simulink model "pocketcorr2"  (Simulink 6.2)
settings: Solver=ode45  StartTime=0.0  StopTime=1000  RelTol=1e-3
libraries: xbsIndex_r3 x143, xps_library x15, ddc_library x9, cic_library x4, fft_library x3, correlator_library x3, pfb_library x2, delay_lib x1
(part 1 of 2)
settings Model: LastModifiedBy=dejesusc
settings DebuggingCC: SolverPrmCheckMsg=warning

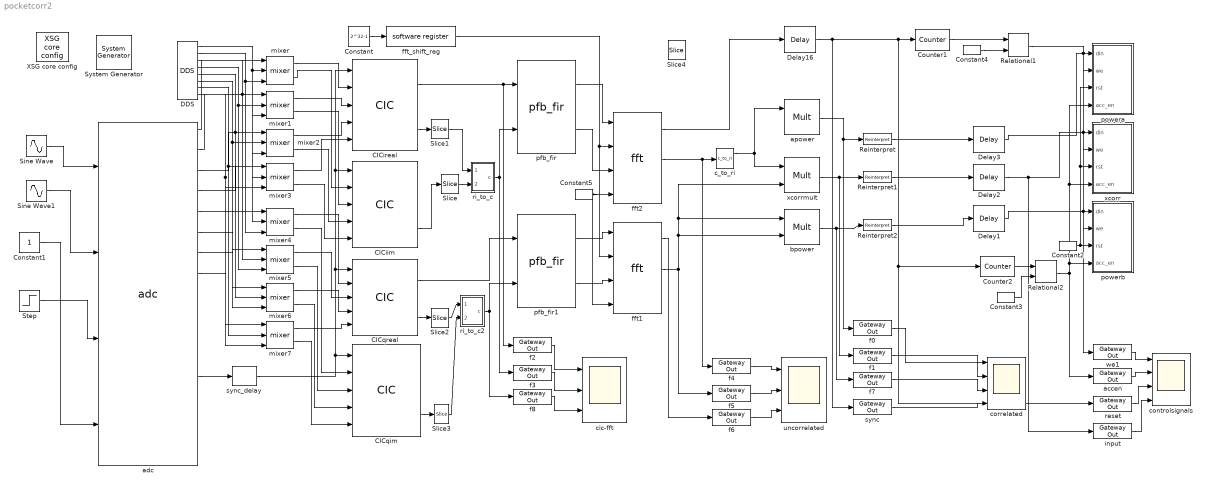
== system pocketcorr2 ==
  " System Generator" : xbsIndex_r3/ System Generator  Tag=genX  xilinxfamily=Virtex2P  part=xc2vp50  speed=-7  package=ff1152  synthesis_tool=XST  directory=./pocketcorr2/sysgen  testbench=off  simulink_period=1  sysclk_period=6.6667  incr_netlist=off  trim_vbits=Everywhere in SubSystem  dbl_ovrd=According to Block Masks  core_generation=According to Block Masks  run_coregen=off  deprecated_control=off  eval_field=0
      settings: AttributesFormatString=System\nGenerator
  CICiim : cic_library/CIC  Description="Cascaded integrator-comb filter.  Linear phase response."  inputs=4  input_bitwidth=16  input_binary_pt=14  D=1  R=1  stages=1  pipeline=off  add_latency=2  int_latency=1  comb_latency=1
  CICireal : cic_library/CIC  Description="Cascaded integrator-comb filter.  Linear phase response."  inputs=4  input_bitwidth=16  input_binary_pt=14  D=1  R=1  stages=1  pipeline=off  add_latency=2  int_latency=1  comb_latency=1
  CICqim : cic_library/CIC  Description="Cascaded integrator-comb filter.  Linear phase response."  inputs=4  input_bitwidth=16  input_binary_pt=14  D=1  R=1  stages=1  pipeline=off  add_latency=2  int_latency=1  comb_latency=1
  CICqreal : cic_library/CIC  Description="Cascaded integrator-comb filter.  Linear phase response."  inputs=4  input_bitwidth=16  input_binary_pt=14  D=1  R=1  stages=1  pipeline=off  add_latency=2  int_latency=1  comb_latency=1
  Constant : Constant  Value=2^32-1
  Constant1 : Constant
  Constant2 : xbsIndex_r3/Constant  const=0  equ=P=C  arith_type=Boolean  n_bits=1  bin_pt=0  opselect=C  inp2=PCIN>>17  opr=+  inp1=P  carry=CIN  iostate=0  explicit_period=on  period=1  dbl_ovrd=off
  Constant3 : xbsIndex_r3/Constant  const=64  equ=P=C  arith_type=Unsigned  n_bits=7  bin_pt=0  opselect=C  inp2=PCIN>>17  opr=+  inp1=P  carry=CIN  iostate=0  explicit_period=on  period=1  dbl_ovrd=off
  Constant4 : xbsIndex_r3/Constant  const=2^4  equ=P=C  arith_type=Unsigned  n_bits=6  bin_pt=0  opselect=C  inp2=PCIN>>17  opr=+  inp1=P  carry=CIN  iostate=0  explicit_period=on  period=1  dbl_ovrd=off
  Constant5 : xbsIndex_r3/Constant  const=0  equ=P=C  arith_type=Unsigned  n_bits=1  bin_pt=0  opselect=C  inp2=PCIN>>17  opr=+  inp1=P  carry=CIN  iostate=0  explicit_period=on  period=1  dbl_ovrd=off
  Counter1 : xbsIndex_r3/Counter  cnt_type=Free Running  n_bits=5  bin_pt=0  arith_type=Unsigned  start_count=0  cnt_to=Inf  cnt_by_val=1  operation=Up  explicit_period=off  period=1  load_pin=off  rst=on  en=off  dbl_ovrd=off  show_param=off  use_rpm=on  gen_core=off
      settings: xl_area=[0, 0, 0, 0, 0, 0, 0]
  Counter2 : xbsIndex_r3/Counter  cnt_type=Free Running  n_bits=8  bin_pt=0  arith_type=Unsigned  start_count=0  cnt_to=Inf  cnt_by_val=1  operation=Up  explicit_period=off  period=1  load_pin=off  rst=on  en=off  dbl_ovrd=off  show_param=off  use_rpm=on  gen_core=off
      settings: xl_area=[0, 0, 0, 0, 0, 0, 0]
  DDS : ddc_library/DDS  freq_div=8  freq=2  num_lo=4  BitWidth=8  latency=2
      link override ddc_lo0/ddc_lo_const/const: equ=P=C
      link override ddc_lo0/ddc_lo_const/const1: equ=P=C
      link override ddc_lo1/ddc_lo_const/const: equ=P=C
      link override ddc_lo1/ddc_lo_const/const1: equ=P=C
      link override ddc_lo2/ddc_lo_const/const: equ=P=C
      link override ddc_lo2/ddc_lo_const/const1: equ=P=C
      link override ddc_lo3/ddc_lo_const/const: equ=P=C
      link override ddc_lo3/ddc_lo_const/const1: equ=P=C
  Delay1 : xbsIndex_r3/Delay  latency=1  reg_retiming=off  explicit_period=on  period=1  en=off  accept_only_valid=off  init_zero=on  dbl_ovrd=off  show_param=off
      settings: xl_area=[0, 0, 0, 0, 0, 0, 0]
  Delay16 : xbsIndex_r3/Delay  latency=5  reg_retiming=off  explicit_period=on  period=1  en=off  accept_only_valid=off  init_zero=on  dbl_ovrd=off  show_param=off
      settings: xl_area=[0, 0, 0, 0, 0, 0, 0]
  Delay2 : xbsIndex_r3/Delay  latency=1  reg_retiming=off  explicit_period=on  period=1  en=off  accept_only_valid=off  init_zero=on  dbl_ovrd=off  show_param=off
      settings: xl_area=[0, 0, 0, 0, 0, 0, 0]
  Delay3 : xbsIndex_r3/Delay  latency=1  reg_retiming=off  explicit_period=on  period=1  en=off  accept_only_valid=off  init_zero=on  dbl_ovrd=off  show_param=off
      settings: xl_area=[0, 0, 0, 0, 0, 0, 0]
  Reinterpret : xbsIndex_r3/Reinterpret  force_arith_type=on  arith_type=Unsigned  force_bin_pt=on  bin_pt=20  force_valid=on
  Reinterpret1 : xbsIndex_r3/Reinterpret  force_arith_type=on  arith_type=Unsigned  force_bin_pt=on  bin_pt=20  force_valid=on
  Reinterpret2 : xbsIndex_r3/Reinterpret  force_arith_type=on  arith_type=Unsigned  force_bin_pt=on  bin_pt=20  force_valid=on
  Relational1 : xbsIndex_r3/Relational  mode=a<b  latency=1  explicit_period=on  period=1  en=off  dbl_ovrd=off  show_param=off
      settings: xl_area=[0, 0, 0, 0, 0, 0, 0]
  Relational2 : xbsIndex_r3/Relational  mode=a<b  latency=1  explicit_period=on  period=1  en=off  dbl_ovrd=off  show_param=off
      settings: xl_area=[0, 0, 0, 0, 0, 0, 0]
  Sine Wave : Sin  SampleTime=0
  Sine Wave1 : Sin  Frequency=2  SampleTime=0
  Slice{,1..4} (5 alike) : xbsIndex_r3/Slice  mode=Upper Bit Location + Width  nbits=9  bit1=0  base1=MSB of Input  bit0=0  base0=LSB of Input  boolean_output=off  explicit_period=off  period=1  dbl_ovrd=off
  Step : Step  Time=10  Before=1  After=0  SampleTime=0
  XSG core config : xps_library/XSG core config  Tag=xps:xsg  hw_sys=iBOB  clk_src=adc0_clk  clk_rate=150  sample_period=1  synthesis_tool=XST  mpc_type=powerpc405
  accen : xbsIndex_r3/Gateway Out  output_type=Double  nbits=8  bin_pt=6  arith_type=Boolean  quantization=Truncate  overflow=Wrap  hdl_port=on  timing_constraint=None  locs_specified=off  LOCs={}  needs_fixed_name=off  show_param=off
      settings: xl_area=[0, 0, 0, 0, 0, 0, 0]
  adc : xps_library/adc  Tag=xps:adc  adc_brd=iBOB:adc0  adc_clk_rate=600  adc_interleave=off  sample_period=1
  apower : xbsIndex_r3/Mult  precision=Full  arith_type="Signed  (2's comp)"  n_bits=8  bin_pt=2  quantization=Truncate  overflow=Wrap  latency=5  explicit_period=on  period=1  en=off  dbl_ovrd=off  show_param=off  mult_type=Parallel  oversample=2  use_embedded=off  pipeline=on  use_rpm=on  placement_style=Rectangular Shape  gen_core=off
      settings: xl_area=[0, 0, 0, 0, 0, 0, 0]
  bpower : xbsIndex_r3/Mult  precision=Full  arith_type="Signed  (2's comp)"  n_bits=8  bin_pt=2  quantization=Truncate  overflow=Wrap  latency=5  explicit_period=on  period=1  en=off  dbl_ovrd=off  show_param=off  mult_type=Parallel  oversample=2  use_embedded=off  pipeline=on  use_rpm=on  placement_style=Rectangular Shape  gen_core=off
      settings: xl_area=[0, 0, 0, 0, 0, 0, 0]
  c_to_ri : fft_library/c_to_ri  BitWidth=18
  cic-fft : Scope  NumInputPorts=3
      settings: YMin=-5~-5~-5  YMax=5~5~5  SaveName=ScopeData3
  controlsignals : Scope  NumInputPorts=4
      settings: YMin=-5~-5~-5~-5  YMax=5~5~5~5  SaveName=ScopeData4
  correlated : Scope  NumInputPorts=4
      settings: YMin=-5~-5~-5~-5  YMax=5~5~5~5
  f{0..1,3..8} (8 alike) : xbsIndex_r3/Gateway Out  output_type=Double  nbits=8  bin_pt=6  arith_type=Boolean  quantization=Truncate  overflow=Wrap  hdl_port=on  timing_constraint=None  locs_specified=off  LOCs={}  needs_fixed_name=off  show_param=off
      settings: xl_area=[0, 0, 0, 0, 0, 0, 0]
  f2 : xbsIndex_r3/Gateway Out  output_type=Automatic  nbits=8  bin_pt=6  arith_type=Boolean  quantization=Truncate  overflow=Wrap  hdl_port=on  timing_constraint=None  locs_specified=off  LOCs={}  needs_fixed_name=off  show_param=off
      settings: xl_area=[0, 0, 0, 0, 0, 0, 0]
  fft1 : fft_library/fft  FFTSize=5  BitWidth=72  n_inputs=0  quantization=Truncate  overflow=Wrap  add_latency=2  mult_latency=3  bram_latency=2
  fft2 : fft_library/fft  FFTSize=5  BitWidth=72  n_inputs=0  quantization=Truncate  overflow=Wrap  add_latency=2  mult_latency=3  bram_latency=2
  fft_shift_reg : xps_library/software register  Tag=xps:sw_reg  io_dir=From Processor  arith_type=Unsigned  bitwidth=32  bin_pt=0  sample_period=1  gw_name=pocketcorr2_fft_shift_reg_user_data_out
  input : xbsIndex_r3/Gateway Out  output_type=Double  nbits=8  bin_pt=6  arith_type=Boolean  quantization=Truncate  overflow=Wrap  hdl_port=on  timing_constraint=None  locs_specified=off  LOCs={}  needs_fixed_name=off  show_param=off
      settings: xl_area=[0, 0, 0, 0, 0, 0, 0]
  mixer{,1..7} (8 alike) : ddc_library/mixer  BitWidth=18  latency=2
  pfb_fir : pfb_library/pfb_fir  PFBSize=5  TotalTaps=2  WindowType=hamming  n_inputs=0  MakeBiplex=off  BitWidthIn=18  BitWidthOut=36  CoeffBitWidth=8  CoeffDistMem=off  add_latency=2  mult_latency=3  bram_latency=2  quantization="Round  (unbiased: +/- Inf)"  fwidth=1
      link override pol1_in1_first_tap/sync_delay/Constant: equ=P=C
      link override pol1_in1_first_tap/sync_delay/Constant1: equ=P=C
      link override pol1_in1_first_tap/sync_delay/Constant2: equ=P=C
      link override pol1_in1_first_tap/sync_delay/Constant3: equ=P=C
  pfb_fir1 : pfb_library/pfb_fir  PFBSize=5  TotalTaps=2  WindowType=hamming  n_inputs=0  MakeBiplex=off  BitWidthIn=18  BitWidthOut=36  CoeffBitWidth=8  CoeffDistMem=off  add_latency=2  mult_latency=3  bram_latency=2  quantization="Round  (unbiased: +/- Inf)"  fwidth=1
      link override pol1_in1_first_tap/sync_delay/Constant: equ=P=C
      link override pol1_in1_first_tap/sync_delay/Constant1: equ=P=C
      link override pol1_in1_first_tap/sync_delay/Constant2: equ=P=C
      link override pol1_in1_first_tap/sync_delay/Constant3: equ=P=C
  powera : Subsystem  AncestorBlock=correlator_library/vacc  mask{vlen=32/2-1, n_bits=32, bin_pt=0, add_latency=2, arith_type=Unsigned, BitWidthIn=72, BinPtIn=20, streams=1}
      mask prompts: vlen "Vector Length"; n_bits "Output Sample Bit Width"; bin_pt "Output Binary Point"; add_latency "Add Latency"; arith_type "Arithmetic Type"; BitWidthIn "Input Bit Width"; BinPtIn "Input Binary Point"; streams "Number of Parallel Streams"
      mask init:
      | cursys = gcb;
      | disp(cursys);
      | 
      | core = [cursys,'/acc_core'];
      | if ~strcmp(get_param(core, 'arith_type'), arith_type),
      |     set_param(core, 'arith_type', arith_type);
      | end
      mask StyleString: edit,edit,edit,edit,popup(Unsigned|Signed  (2's comp)),edit,edit,edit
  powerb : Subsystem  AncestorBlock=correlator_library/vacc  mask{vlen=32/2-1, n_bits=32, bin_pt=0, add_latency=2, arith_type=Unsigned, BitWidthIn=72, BinPtIn=20, streams=1}
      mask prompts: vlen "Vector Length"; n_bits "Output Sample Bit Width"; bin_pt "Output Binary Point"; add_latency "Add Latency"; arith_type "Arithmetic Type"; BitWidthIn "Input Bit Width"; BinPtIn "Input Binary Point"; streams "Number of Parallel Streams"
      mask init:
      | cursys = gcb;
      | disp(cursys);
      | 
      | core = [cursys,'/acc_core'];
      | if ~strcmp(get_param(core, 'arith_type'), arith_type),
      |     set_param(core, 'arith_type', arith_type);
      | end
      mask StyleString: edit,edit,edit,edit,popup(Unsigned|Signed  (2's comp)),edit,edit,edit
  reset : xbsIndex_r3/Gateway Out  output_type=Double  nbits=8  bin_pt=6  arith_type=Boolean  quantization=Truncate  overflow=Wrap  hdl_port=on  timing_constraint=None  locs_specified=off  LOCs={}  needs_fixed_name=off  show_param=off
      settings: xl_area=[0, 0, 0, 0, 0, 0, 0]
  ri_to_c : Subsystem  AncestorBlock=fft_library/ri_to_c  mask{likes_cookies=on}
      mask prompts: likes_cookies "I think cookies are delicious"
  ri_to_c2 : Subsystem  AncestorBlock=fft_library/ri_to_c  mask{likes_cookies=on}
      mask prompts: likes_cookies "I think cookies are delicious"
  sync : xbsIndex_r3/Gateway Out  output_type=Double  nbits=8  bin_pt=6  arith_type=Boolean  quantization=Truncate  overflow=Wrap  hdl_port=on  timing_constraint=None  locs_specified=off  LOCs={}  needs_fixed_name=off  show_param=off
      settings: xl_area=[0, 0, 0, 0, 0, 0, 0]
  sync_delay : delay_lib/sync_delay  DelayLen=4
      link override Constant: equ=P=C
      link override Constant1: equ=P=C
      link override Constant2: equ=P=C
      link override Constant3: equ=P=C
  uncorrelated : Scope  NumInputPorts=3
      settings: YMin=-5~-5~-5  YMax=5~5~5  SaveName=ScopeData2
  we1 : xbsIndex_r3/Gateway Out  output_type=Double  nbits=8  bin_pt=6  arith_type=Boolean  quantization=Truncate  overflow=Wrap  hdl_port=on  timing_constraint=None  locs_specified=off  LOCs={}  needs_fixed_name=off  show_param=off
      settings: xl_area=[0, 0, 0, 0, 0, 0, 0]
  xcorr : Subsystem  AncestorBlock=correlator_library/vacc  mask{vlen=32/2-1, n_bits=32, bin_pt=0, add_latency=2, arith_type=Unsigned, BitWidthIn=72, BinPtIn=20, streams=1}
      mask prompts: vlen "Vector Length"; n_bits "Output Sample Bit Width"; bin_pt "Output Binary Point"; add_latency "Add Latency"; arith_type "Arithmetic Type"; BitWidthIn "Input Bit Width"; BinPtIn "Input Binary Point"; streams "Number of Parallel Streams"
      mask init:
      | cursys = gcb;
      | disp(cursys);
      | 
      | core = [cursys,'/acc_core'];
      | if ~strcmp(get_param(core, 'arith_type'), arith_type),
      |     set_param(core, 'arith_type', arith_type);
      | end
      mask StyleString: edit,edit,edit,edit,popup(Unsigned|Signed  (2's comp)),edit,edit,edit
  xcorrmult : xbsIndex_r3/Mult  precision=Full  arith_type="Signed  (2's comp)"  n_bits=8  bin_pt=2  quantization=Truncate  overflow=Wrap  latency=5  explicit_period=on  period=1  en=off  dbl_ovrd=off  show_param=off  mult_type=Parallel  oversample=2  use_embedded=off  pipeline=on  use_rpm=on  placement_style=Rectangular Shape  gen_core=off
      settings: xl_area=[0, 0, 0, 0, 0, 0, 0]
  wires:
  Constant/1 -> fft_shift_reg/1
  Constant1/1 -> adc/4
  apower/1 -> f0/1, Reinterpret/1
  xcorrmult/1 -> f1/1, Reinterpret1/1
  Delay16/1 -> Counter1/1, Counter2/1, reset/1, sync/1
  Step/1 -> adc/3
  Sine Wave/1 -> adc/1
  Counter1/1 -> Relational1/1
  Constant4/1 -> Relational1/2
  Relational1/1 -> powera/2(we), powerb/2(we), we1/1, xcorr/2(we)
  Constant2/1 -> powerb/3(rst), xcorr/3(rst), powera/3(rst)
  Relational2/1 -> accen/1, powerb/4(acc_en), xcorr/4(acc_en), powera/4(acc_en)
  Counter2/1 -> Relational2/1
  Constant3/1 -> Relational2/2
  f0/1 -> correlated/1
  f1/1 -> correlated/2
  f4/1 -> uncorrelated/1
  f5/1 -> uncorrelated/2
  f6/1 -> uncorrelated/3
  DDS/1 -> mixer/2, mixer4/2
  DDS/2 -> mixer/3, mixer4/3
  adc/1 -> mixer/1
  DDS/3 -> mixer1/2, mixer5/2
  DDS/4 -> mixer1/3, mixer5/3
  DDS/5 -> mixer2/2, mixer6/2
  DDS/6 -> mixer2/3, mixer6/3
  adc/2 -> mixer1/1
  adc/3 -> mixer2/1
  adc/4 -> mixer3/1
  adc/5 -> mixer4/1
  adc/6 -> mixer5/1
  adc/7 -> mixer6/1
  adc/8 -> mixer7/1
  DDS/7 -> mixer3/2, mixer7/2
  DDS/8 -> mixer3/3, mixer7/3
  adc/13 -> sync_delay/1
  bpower/1 -> Reinterpret2/1, f7/1
  fft_shift_reg/1 -> fft2/2, fft1/2
  fft2/1 -> Delay16/1
  fft1/2 -> xcorrmult/2, bpower/1, bpower/2, f5/1
  fft2/2 -> f4/1, c_to_ri/1
  fft1/1 -> f6/1
  sync/1 -> correlated/4
  f7/1 -> correlated/3
  CICireal/2 -> Slice1/1
  CICiim/2 -> Slice/1
  CICqreal/2 -> Slice2/1
  CICqim/2 -> Slice3/1
  ri_to_c2/1(c) -> f8/1, pfb_fir1/2
  ri_to_c/1(c) -> f3/1, pfb_fir/2
  CICireal/1 -> f2/1, pfb_fir/1
  f2/1 -> cic-fft/1
  f3/1 -> cic-fft/2
  f8/1 -> cic-fft/3
  Constant5/1 -> fft2/4, fft1/4
  Slice/1 -> ri_to_c/2(im)
  Slice1/1 -> ri_to_c/1(re)
  Slice2/1 -> ri_to_c2/1(re)
  Slice3/1 -> ri_to_c2/2(im)
  we1/1 -> controlsignals/1
  accen/1 -> controlsignals/2
  reset/1 -> controlsignals/3
  input/1 -> controlsignals/4
  Delay1/1 -> powerb/1(din)
  Reinterpret/1 -> Delay3/1
  Reinterpret1/1 -> Delay2/1
  Reinterpret2/1 -> Delay1/1
  Delay2/1 -> xcorr/1(din), input/1
  Delay3/1 -> powera/1(din)
  sync_delay/1 -> CICqim/1, CICqreal/1, CICiim/1, CICireal/1
  mixer/1 -> CICireal/2
  mixer/2 -> CICiim/2
  mixer1/1 -> CICireal/3
  mixer1/2 -> CICiim/3
  mixer2/1 -> CICireal/4
  mixer2/2 -> CICiim/4
  mixer3/1 -> CICireal/5
  mixer3/2 -> CICiim/5
  mixer4/1 -> CICqreal/2
  mixer5/1 -> CICqreal/3
  mixer6/1 -> CICqreal/4
  mixer7/1 -> CICqreal/5
  mixer4/2 -> CICqim/2
  mixer5/2 -> CICqim/3
  mixer6/2 -> CICqim/4
  mixer7/2 -> CICqim/5
  pfb_fir1/2 -> fft1/3
  pfb_fir1/1 -> fft1/1
  CICqreal/1 -> pfb_fir1/1
  pfb_fir/2 -> fft2/3
  pfb_fir/1 -> fft2/1
  Sine Wave1/1 -> adc/2
  c_to_ri/1 -> apower/1, xcorrmult/1

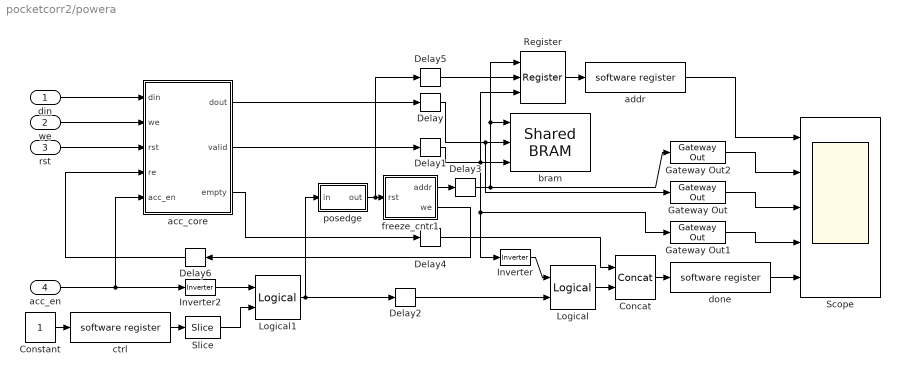
== system pocketcorr2/powera ==
  din : Inport  Port=1  LatchInput=off
  we : Inport  Port=2  LatchInput=off
  rst : Inport  Port=3  LatchInput=off
  acc_en : Inport  Port=4  LatchInput=off
  Concat : xbsIndex_r3/Concat  num_inputs=2  explicit_period=off  period=1  dbl_ovrd=off
  Constant : Constant
  Delay : xbsIndex_r3/Delay  latency=1  reg_retiming=off  explicit_period=off  period=1  en=off  accept_only_valid=off  init_zero=on  dbl_ovrd=off  show_param=off
      settings: xl_area=[0, 0, 0, 0, 0, 0, 0]
  Delay1 : xbsIndex_r3/Delay  latency=1  reg_retiming=off  explicit_period=off  period=1  en=off  accept_only_valid=off  init_zero=on  dbl_ovrd=off  show_param=off
      settings: xl_area=[0, 0, 0, 0, 0, 0, 0]
  Delay2 : xbsIndex_r3/Delay  latency=6  reg_retiming=off  explicit_period=off  period=1  en=off  accept_only_valid=off  init_zero=on  dbl_ovrd=off  show_param=off
      settings: xl_area=[0, 0, 0, 0, 0, 0, 0]
  Delay3 : xbsIndex_r3/Delay  latency=4  reg_retiming=off  explicit_period=off  period=1  en=off  accept_only_valid=off  init_zero=on  dbl_ovrd=off  show_param=off
      settings: xl_area=[0, 0, 0, 0, 0, 0, 0]
  Delay4 : xbsIndex_r3/Delay  latency=2  reg_retiming=off  explicit_period=on  period=1  en=off  accept_only_valid=off  init_zero=on  dbl_ovrd=off  show_param=off
      settings: xl_area=[0, 0, 0, 0, 0, 0, 0]
  Delay5 : xbsIndex_r3/Delay  latency=3  reg_retiming=off  explicit_period=off  period=1  en=off  accept_only_valid=off  init_zero=on  dbl_ovrd=off  show_param=off
      settings: xl_area=[0, 0, 0, 0, 0, 0, 0]
  Delay6 : xbsIndex_r3/Delay  Orientation=left  latency=3  reg_retiming=off  explicit_period=off  period=1  en=off  accept_only_valid=off  init_zero=on  dbl_ovrd=off  show_param=off
      settings: xl_area=[0, 0, 0, 0, 0, 0, 0]
  Gateway Out : xbsIndex_r3/Gateway Out  output_type=Double  nbits=8  bin_pt=6  arith_type=Boolean  quantization=Truncate  overflow=Wrap  hdl_port=off  timing_constraint=None  locs_specified=off  LOCs={}  needs_fixed_name=off  show_param=off
      settings: xl_area=[0, 0, 0, 0, 0, 0, 0]
  Gateway Out1 : xbsIndex_r3/Gateway Out  output_type=Double  nbits=8  bin_pt=6  arith_type=Boolean  quantization=Truncate  overflow=Wrap  hdl_port=off  timing_constraint=None  locs_specified=off  LOCs={}  needs_fixed_name=off  show_param=off
      settings: xl_area=[0, 0, 0, 0, 0, 0, 0]
  Gateway Out2 : xbsIndex_r3/Gateway Out  output_type=Double  nbits=8  bin_pt=6  arith_type=Boolean  quantization=Truncate  overflow=Wrap  hdl_port=off  timing_constraint=None  locs_specified=off  LOCs={}  needs_fixed_name=off  show_param=off
      settings: xl_area=[0, 0, 0, 0, 0, 0, 0]
  Inverter : xbsIndex_r3/Inverter  latency=0  explicit_period=off  period=1  en=off  dbl_ovrd=off  show_param=off
      settings: xl_area=[0, 0, 0, 0, 0, 0, 0]
  Inverter2 : xbsIndex_r3/Inverter  latency=0  explicit_period=off  period=1  en=off  dbl_ovrd=off  show_param=off
      settings: xl_area=[0, 0, 0, 0, 0, 0, 0]
  Logical : xbsIndex_r3/Logical  logical_function=AND  inputs=2  precision=Full  arith_type=Unsigned  n_bits=8  bin_pt=2  align_bp=on  latency=0  explicit_period=off  period=1  en=off  dbl_ovrd=off  show_param=off
      settings: xl_area=[0, 0, 0, 0, 0, 0, 0]
  Logical1 : xbsIndex_r3/Logical  logical_function=AND  inputs=2  precision=Full  arith_type=Unsigned  n_bits=8  bin_pt=2  align_bp=on  latency=1  explicit_period=off  period=1  en=off  dbl_ovrd=off  show_param=off
      settings: xl_area=[0, 0, 0, 0, 0, 0, 0]
  Register : xbsIndex_r3/Register  init=0  reg_only_valid=off  explicit_period=off  period=1  rst=on  en=on  out_en=off  dbl_ovrd=off  show_param=off
      settings: xl_area=[0, 0, 0, 0, 0, 0, 0]
  Scope : Scope  NumInputPorts=5
      settings: YMin=0~0~0~0~0  YMax=50~200~4~1~3
  Slice : xbsIndex_r3/Slice  mode=Lower Bit Location + Width  nbits=1  bit1=0  base1=MSB of Input  bit0=0  base0=LSB of Input  boolean_output=on  explicit_period=off  period=1  dbl_ovrd=off
  acc_core : Subsystem  mask{vlen=vlen, n_bits=n_bits, bin_pt=bin_pt, add_latency=add_latency, arith_type=Unsigned, BitWidthIn=BitWidthIn, BinPtIn=BinPtIn, streams=streams}
      mask prompts: vlen "Vector Length"; n_bits "Output Sample Bit Width"; bin_pt "Output Binary Point"; add_latency "Add Latency"; arith_type "Arithmetic Type"; BitWidthIn "Input Bit Width"; BinPtIn "Input Binary Point"; streams "Number of Parallel Streams"
      mask init:
      | acc_core_mask;
      mask StyleString: edit,edit,edit,edit,popup(Unsigned|Signed  (2's comp)),edit,edit,edit
  addr : xps_library/software register  Tag=xps:sw_reg  io_dir=To Processor  arith_type=Unsigned  bitwidth=32  bin_pt=0  sample_period=1  gw_name=pocketcorr2_powera_addr_user_data_in
  bram : xps_library/Shared BRAM  Tag=xps:bram  arith_type="Signed  (2's comp)"  addr_width=11  data_width=32  data_bin_pt=bin_pt  init_vals=0  sample_rate=1
  ctrl : xps_library/software register  Tag=xps:sw_reg  io_dir=From Processor  arith_type=Unsigned  bitwidth=32  bin_pt=0  sample_period=1  gw_name=pocketcorr2_powera_ctrl_user_data_out
  done : xps_library/software register  Tag=xps:sw_reg  io_dir=To Processor  arith_type=Unsigned  bitwidth=32  bin_pt=0  sample_period=1  gw_name=pocketcorr2_powera_done_user_data_in
  freeze_cntr1 : Subsystem  mask{CounterBits=11}
      mask prompts: CounterBits "Counter Length (2^?)"
  posedge : Subsystem
  wires:
  Delay5/1 -> Register/2
  Delay6/1 -> acc_core/4(re)
  Delay4/1 -> Concat/1
  Concat/1 -> done/1
  Logical/1 -> Concat/2
  acc_core/3(empty) -> Delay4/1
  Register/1 -> addr/1
  Delay3/1 -> Register/1, bram/1, Gateway Out2/1
  Delay2/1 -> Logical/2
  Delay1/1 -> Register/3, bram/3, Inverter/1, Gateway Out1/1
  Constant/1 -> ctrl/1
  Delay/1 -> Gateway Out/1, bram/2
  din/1 -> acc_core/1(din)
  we/1 -> acc_core/2(we)
  rst/1 -> acc_core/3(rst)
  acc_core/2(valid) -> Delay1/1
  freeze_cntr1/1(addr) -> Delay3/1
  freeze_cntr1/2(we) -> Delay6/1
  acc_core/1(dout) -> Delay/1
  Inverter/1 -> Logical/1
  acc_en/1 -> acc_core/5(acc_en), Inverter2/1
  ctrl/1 -> Slice/1
  Slice/1 -> Logical1/2
  Inverter2/1 -> Logical1/1
  Logical1/1 -> Delay2/1, posedge/1(in)
  posedge/1(out) -> Delay5/1, freeze_cntr1/1(rst)
  done/1 -> Scope/5
  Gateway Out1/1 -> Scope/4
  Gateway Out/1 -> Scope/3
  addr/1 -> Scope/1
  Gateway Out2/1 -> Scope/2

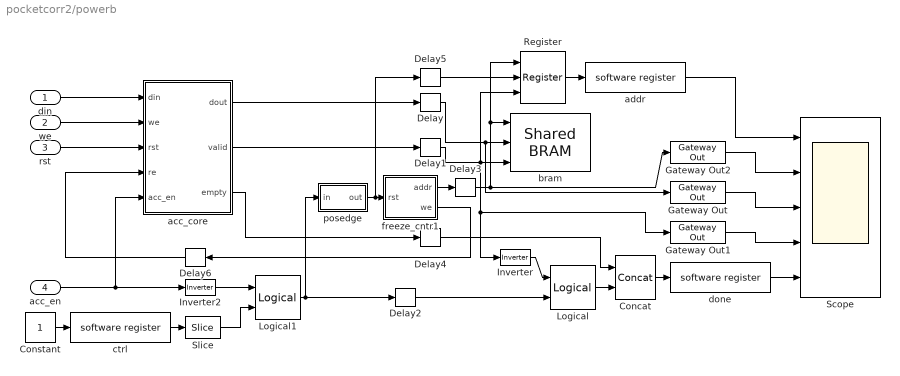
== system pocketcorr2/powerb ==
  din : Inport  Port=1  LatchInput=off
  we : Inport  Port=2  LatchInput=off
  rst : Inport  Port=3  LatchInput=off
  acc_en : Inport  Port=4  LatchInput=off
  Concat : xbsIndex_r3/Concat  num_inputs=2  explicit_period=off  period=1  dbl_ovrd=off
  Constant : Constant
  Delay : xbsIndex_r3/Delay  latency=1  reg_retiming=off  explicit_period=off  period=1  en=off  accept_only_valid=off  init_zero=on  dbl_ovrd=off  show_param=off
      settings: xl_area=[0, 0, 0, 0, 0, 0, 0]
  Delay1 : xbsIndex_r3/Delay  latency=1  reg_retiming=off  explicit_period=off  period=1  en=off  accept_only_valid=off  init_zero=on  dbl_ovrd=off  show_param=off
      settings: xl_area=[0, 0, 0, 0, 0, 0, 0]
  Delay2 : xbsIndex_r3/Delay  latency=6  reg_retiming=off  explicit_period=off  period=1  en=off  accept_only_valid=off  init_zero=on  dbl_ovrd=off  show_param=off
      settings: xl_area=[0, 0, 0, 0, 0, 0, 0]
  Delay3 : xbsIndex_r3/Delay  latency=4  reg_retiming=off  explicit_period=off  period=1  en=off  accept_only_valid=off  init_zero=on  dbl_ovrd=off  show_param=off
      settings: xl_area=[0, 0, 0, 0, 0, 0, 0]
  Delay4 : xbsIndex_r3/Delay  latency=2  reg_retiming=off  explicit_period=on  period=1  en=off  accept_only_valid=off  init_zero=on  dbl_ovrd=off  show_param=off
      settings: xl_area=[0, 0, 0, 0, 0, 0, 0]
  Delay5 : xbsIndex_r3/Delay  latency=3  reg_retiming=off  explicit_period=off  period=1  en=off  accept_only_valid=off  init_zero=on  dbl_ovrd=off  show_param=off
      settings: xl_area=[0, 0, 0, 0, 0, 0, 0]
  Delay6 : xbsIndex_r3/Delay  Orientation=left  latency=3  reg_retiming=off  explicit_period=off  period=1  en=off  accept_only_valid=off  init_zero=on  dbl_ovrd=off  show_param=off
      settings: xl_area=[0, 0, 0, 0, 0, 0, 0]
  Gateway Out : xbsIndex_r3/Gateway Out  output_type=Double  nbits=8  bin_pt=6  arith_type=Boolean  quantization=Truncate  overflow=Wrap  hdl_port=off  timing_constraint=None  locs_specified=off  LOCs={}  needs_fixed_name=off  show_param=off
      settings: xl_area=[0, 0, 0, 0, 0, 0, 0]
  Gateway Out1 : xbsIndex_r3/Gateway Out  output_type=Double  nbits=8  bin_pt=6  arith_type=Boolean  quantization=Truncate  overflow=Wrap  hdl_port=off  timing_constraint=None  locs_specified=off  LOCs={}  needs_fixed_name=off  show_param=off
      settings: xl_area=[0, 0, 0, 0, 0, 0, 0]
  Gateway Out2 : xbsIndex_r3/Gateway Out  output_type=Double  nbits=8  bin_pt=6  arith_type=Boolean  quantization=Truncate  overflow=Wrap  hdl_port=off  timing_constraint=None  locs_specified=off  LOCs={}  needs_fixed_name=off  show_param=off
      settings: xl_area=[0, 0, 0, 0, 0, 0, 0]
  Inverter : xbsIndex_r3/Inverter  latency=0  explicit_period=off  period=1  en=off  dbl_ovrd=off  show_param=off
      settings: xl_area=[0, 0, 0, 0, 0, 0, 0]
  Inverter2 : xbsIndex_r3/Inverter  latency=0  explicit_period=off  period=1  en=off  dbl_ovrd=off  show_param=off
      settings: xl_area=[0, 0, 0, 0, 0, 0, 0]
  Logical : xbsIndex_r3/Logical  logical_function=AND  inputs=2  precision=Full  arith_type=Unsigned  n_bits=8  bin_pt=2  align_bp=on  latency=0  explicit_period=off  period=1  en=off  dbl_ovrd=off  show_param=off
      settings: xl_area=[0, 0, 0, 0, 0, 0, 0]
  Logical1 : xbsIndex_r3/Logical  logical_function=AND  inputs=2  precision=Full  arith_type=Unsigned  n_bits=8  bin_pt=2  align_bp=on  latency=1  explicit_period=off  period=1  en=off  dbl_ovrd=off  show_param=off
      settings: xl_area=[0, 0, 0, 0, 0, 0, 0]
  Register : xbsIndex_r3/Register  init=0  reg_only_valid=off  explicit_period=off  period=1  rst=on  en=on  out_en=off  dbl_ovrd=off  show_param=off
      settings: xl_area=[0, 0, 0, 0, 0, 0, 0]
  Scope : Scope  NumInputPorts=5
      settings: YMin=0~0~0~0~0  YMax=50~200~4~1~3
  Slice : xbsIndex_r3/Slice  mode=Lower Bit Location + Width  nbits=1  bit1=0  base1=MSB of Input  bit0=0  base0=LSB of Input  boolean_output=on  explicit_period=off  period=1  dbl_ovrd=off
  acc_core : Subsystem  mask{vlen=vlen, n_bits=n_bits, bin_pt=bin_pt, add_latency=add_latency, arith_type=Unsigned, BitWidthIn=BitWidthIn, BinPtIn=BinPtIn, streams=streams}
      mask prompts: vlen "Vector Length"; n_bits "Output Sample Bit Width"; bin_pt "Output Binary Point"; add_latency "Add Latency"; arith_type "Arithmetic Type"; BitWidthIn "Input Bit Width"; BinPtIn "Input Binary Point"; streams "Number of Parallel Streams"
      mask init:
      | acc_core_mask;
      mask StyleString: edit,edit,edit,edit,popup(Unsigned|Signed  (2's comp)),edit,edit,edit
  addr : xps_library/software register  Tag=xps:sw_reg  io_dir=To Processor  arith_type=Unsigned  bitwidth=32  bin_pt=0  sample_period=1  gw_name=pocketcorr2_powerb_addr_user_data_in
  bram : xps_library/Shared BRAM  Tag=xps:bram  arith_type="Signed  (2's comp)"  addr_width=11  data_width=32  data_bin_pt=bin_pt  init_vals=0  sample_rate=1
  ctrl : xps_library/software register  Tag=xps:sw_reg  io_dir=From Processor  arith_type=Unsigned  bitwidth=32  bin_pt=0  sample_period=1  gw_name=pocketcorr2_powerb_ctrl_user_data_out
  done : xps_library/software register  Tag=xps:sw_reg  io_dir=To Processor  arith_type=Unsigned  bitwidth=32  bin_pt=0  sample_period=1  gw_name=pocketcorr2_powerb_done_user_data_in
  freeze_cntr1 : Subsystem  mask{CounterBits=11}
      mask prompts: CounterBits "Counter Length (2^?)"
  posedge : Subsystem
  wires:
  Delay5/1 -> Register/2
  Delay6/1 -> acc_core/4(re)
  Delay4/1 -> Concat/1
  Concat/1 -> done/1
  Logical/1 -> Concat/2
  acc_core/3(empty) -> Delay4/1
  Register/1 -> addr/1
  Delay3/1 -> Register/1, bram/1, Gateway Out2/1
  Delay2/1 -> Logical/2
  Delay1/1 -> Register/3, bram/3, Inverter/1, Gateway Out1/1
  Constant/1 -> ctrl/1
  Delay/1 -> Gateway Out/1, bram/2
  din/1 -> acc_core/1(din)
  we/1 -> acc_core/2(we)
  rst/1 -> acc_core/3(rst)
  acc_core/2(valid) -> Delay1/1
  freeze_cntr1/1(addr) -> Delay3/1
  freeze_cntr1/2(we) -> Delay6/1
  acc_core/1(dout) -> Delay/1
  Inverter/1 -> Logical/1
  acc_en/1 -> acc_core/5(acc_en), Inverter2/1
  ctrl/1 -> Slice/1
  Slice/1 -> Logical1/2
  Inverter2/1 -> Logical1/1
  Logical1/1 -> Delay2/1, posedge/1(in)
  posedge/1(out) -> Delay5/1, freeze_cntr1/1(rst)
  done/1 -> Scope/5
  Gateway Out1/1 -> Scope/4
  Gateway Out/1 -> Scope/3
  addr/1 -> Scope/1
  Gateway Out2/1 -> Scope/2

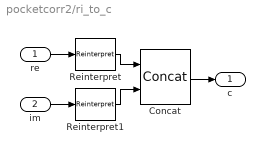
== system pocketcorr2/ri_to_c ==
  re : Inport  Port=1  LatchInput=off
  im : Inport  Port=2  LatchInput=off
  Concat : xbsIndex_r3/Concat  num_inputs=2  explicit_period=on  period=1  dbl_ovrd=off
  Reinterpret : xbsIndex_r3/Reinterpret  force_arith_type=on  arith_type=Unsigned  force_bin_pt=on  bin_pt=0  force_valid=on
  Reinterpret1 : xbsIndex_r3/Reinterpret  force_arith_type=on  arith_type=Unsigned  force_bin_pt=on  bin_pt=0  force_valid=on
  c : Outport
  wires:
  im/1 -> Reinterpret1/1
  Concat/1 -> c/1
  re/1 -> Reinterpret/1
  Reinterpret1/1 -> Concat/2
  Reinterpret/1 -> Concat/1

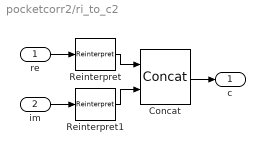
== system pocketcorr2/ri_to_c2 ==
  re : Inport  Port=1  LatchInput=off
  im : Inport  Port=2  LatchInput=off
  Concat : xbsIndex_r3/Concat  num_inputs=2  explicit_period=on  period=1  dbl_ovrd=off
  Reinterpret : xbsIndex_r3/Reinterpret  force_arith_type=on  arith_type=Unsigned  force_bin_pt=on  bin_pt=0  force_valid=on
  Reinterpret1 : xbsIndex_r3/Reinterpret  force_arith_type=on  arith_type=Unsigned  force_bin_pt=on  bin_pt=0  force_valid=on
  c : Outport
  wires:
  im/1 -> Reinterpret1/1
  Concat/1 -> c/1
  re/1 -> Reinterpret/1
  Reinterpret1/1 -> Concat/2
  Reinterpret/1 -> Concat/1

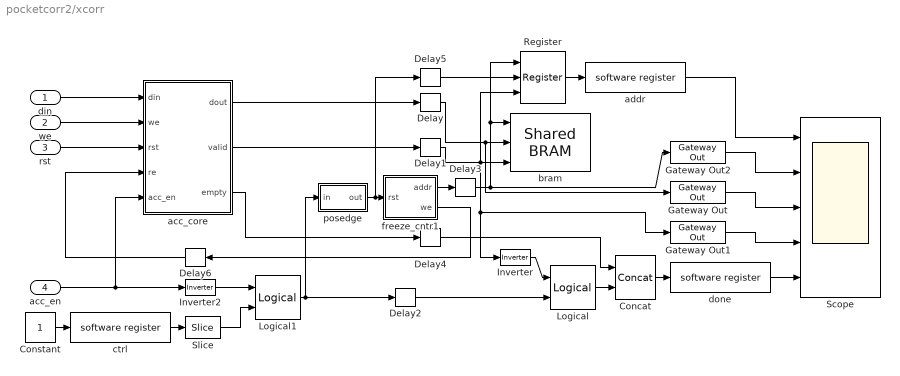
== system pocketcorr2/xcorr ==
  din : Inport  Port=1  LatchInput=off
  we : Inport  Port=2  LatchInput=off
  rst : Inport  Port=3  LatchInput=off
  acc_en : Inport  Port=4  LatchInput=off
  Concat : xbsIndex_r3/Concat  num_inputs=2  explicit_period=off  period=1  dbl_ovrd=off
  Constant : Constant
  Delay : xbsIndex_r3/Delay  latency=1  reg_retiming=off  explicit_period=off  period=1  en=off  accept_only_valid=off  init_zero=on  dbl_ovrd=off  show_param=off
      settings: xl_area=[0, 0, 0, 0, 0, 0, 0]
  Delay1 : xbsIndex_r3/Delay  latency=1  reg_retiming=off  explicit_period=off  period=1  en=off  accept_only_valid=off  init_zero=on  dbl_ovrd=off  show_param=off
      settings: xl_area=[0, 0, 0, 0, 0, 0, 0]
  Delay2 : xbsIndex_r3/Delay  latency=6  reg_retiming=off  explicit_period=off  period=1  en=off  accept_only_valid=off  init_zero=on  dbl_ovrd=off  show_param=off
      settings: xl_area=[0, 0, 0, 0, 0, 0, 0]
  Delay3 : xbsIndex_r3/Delay  latency=4  reg_retiming=off  explicit_period=off  period=1  en=off  accept_only_valid=off  init_zero=on  dbl_ovrd=off  show_param=off
      settings: xl_area=[0, 0, 0, 0, 0, 0, 0]
  Delay4 : xbsIndex_r3/Delay  latency=2  reg_retiming=off  explicit_period=on  period=1  en=off  accept_only_valid=off  init_zero=on  dbl_ovrd=off  show_param=off
      settings: xl_area=[0, 0, 0, 0, 0, 0, 0]
  Delay5 : xbsIndex_r3/Delay  latency=3  reg_retiming=off  explicit_period=off  period=1  en=off  accept_only_valid=off  init_zero=on  dbl_ovrd=off  show_param=off
      settings: xl_area=[0, 0, 0, 0, 0, 0, 0]
  Delay6 : xbsIndex_r3/Delay  Orientation=left  latency=3  reg_retiming=off  explicit_period=off  period=1  en=off  accept_only_valid=off  init_zero=on  dbl_ovrd=off  show_param=off
      settings: xl_area=[0, 0, 0, 0, 0, 0, 0]
  Gateway Out : xbsIndex_r3/Gateway Out  output_type=Double  nbits=8  bin_pt=6  arith_type=Boolean  quantization=Truncate  overflow=Wrap  hdl_port=off  timing_constraint=None  locs_specified=off  LOCs={}  needs_fixed_name=off  show_param=off
      settings: xl_area=[0, 0, 0, 0, 0, 0, 0]
  Gateway Out1 : xbsIndex_r3/Gateway Out  output_type=Double  nbits=8  bin_pt=6  arith_type=Boolean  quantization=Truncate  overflow=Wrap  hdl_port=off  timing_constraint=None  locs_specified=off  LOCs={}  needs_fixed_name=off  show_param=off
      settings: xl_area=[0, 0, 0, 0, 0, 0, 0]
  Gateway Out2 : xbsIndex_r3/Gateway Out  output_type=Double  nbits=8  bin_pt=6  arith_type=Boolean  quantization=Truncate  overflow=Wrap  hdl_port=off  timing_constraint=None  locs_specified=off  LOCs={}  needs_fixed_name=off  show_param=off
      settings: xl_area=[0, 0, 0, 0, 0, 0, 0]
  Inverter : xbsIndex_r3/Inverter  latency=0  explicit_period=off  period=1  en=off  dbl_ovrd=off  show_param=off
      settings: xl_area=[0, 0, 0, 0, 0, 0, 0]
  Inverter2 : xbsIndex_r3/Inverter  latency=0  explicit_period=off  period=1  en=off  dbl_ovrd=off  show_param=off
      settings: xl_area=[0, 0, 0, 0, 0, 0, 0]
  Logical : xbsIndex_r3/Logical  logical_function=AND  inputs=2  precision=Full  arith_type=Unsigned  n_bits=8  bin_pt=2  align_bp=on  latency=0  explicit_period=off  period=1  en=off  dbl_ovrd=off  show_param=off
      settings: xl_area=[0, 0, 0, 0, 0, 0, 0]
  Logical1 : xbsIndex_r3/Logical  logical_function=AND  inputs=2  precision=Full  arith_type=Unsigned  n_bits=8  bin_pt=2  align_bp=on  latency=1  explicit_period=off  period=1  en=off  dbl_ovrd=off  show_param=off
      settings: xl_area=[0, 0, 0, 0, 0, 0, 0]
  Register : xbsIndex_r3/Register  init=0  reg_only_valid=off  explicit_period=off  period=1  rst=on  en=on  out_en=off  dbl_ovrd=off  show_param=off
      settings: xl_area=[0, 0, 0, 0, 0, 0, 0]
  Scope : Scope  NumInputPorts=5
      settings: YMin=0~0~0~0~0  YMax=50~200~4~1~3
  Slice : xbsIndex_r3/Slice  mode=Lower Bit Location + Width  nbits=1  bit1=0  base1=MSB of Input  bit0=0  base0=LSB of Input  boolean_output=on  explicit_period=off  period=1  dbl_ovrd=off
  acc_core : Subsystem  mask{vlen=vlen, n_bits=n_bits, bin_pt=bin_pt, add_latency=add_latency, arith_type=Unsigned, BitWidthIn=BitWidthIn, BinPtIn=BinPtIn, streams=streams}
      mask prompts: vlen "Vector Length"; n_bits "Output Sample Bit Width"; bin_pt "Output Binary Point"; add_latency "Add Latency"; arith_type "Arithmetic Type"; BitWidthIn "Input Bit Width"; BinPtIn "Input Binary Point"; streams "Number of Parallel Streams"
      mask init:
      | acc_core_mask;
      mask StyleString: edit,edit,edit,edit,popup(Unsigned|Signed  (2's comp)),edit,edit,edit
  addr : xps_library/software register  Tag=xps:sw_reg  io_dir=To Processor  arith_type=Unsigned  bitwidth=32  bin_pt=0  sample_period=1  gw_name=pocketcorr2_xcorr_addr_user_data_in
  bram : xps_library/Shared BRAM  Tag=xps:bram  arith_type="Signed  (2's comp)"  addr_width=11  data_width=32  data_bin_pt=bin_pt  init_vals=0  sample_rate=1
  ctrl : xps_library/software register  Tag=xps:sw_reg  io_dir=From Processor  arith_type=Unsigned  bitwidth=32  bin_pt=0  sample_period=1  gw_name=pocketcorr2_xcorr_ctrl_user_data_out
  done : xps_library/software register  Tag=xps:sw_reg  io_dir=To Processor  arith_type=Unsigned  bitwidth=32  bin_pt=0  sample_period=1  gw_name=pocketcorr2_xcorr_done_user_data_in
  freeze_cntr1 : Subsystem  mask{CounterBits=11}
      mask prompts: CounterBits "Counter Length (2^?)"
  posedge : Subsystem
  wires:
  Gateway Out2/1 -> Scope/2
  addr/1 -> Scope/1
  Gateway Out/1 -> Scope/3
  Gateway Out1/1 -> Scope/4
  done/1 -> Scope/5
  posedge/1(out) -> freeze_cntr1/1(rst), Delay5/1
  Logical1/1 -> posedge/1(in), Delay2/1
  Inverter2/1 -> Logical1/1
  Slice/1 -> Logical1/2
  ctrl/1 -> Slice/1
  acc_en/1 -> Inverter2/1, acc_core/5(acc_en)
  Inverter/1 -> Logical/1
  acc_core/1(dout) -> Delay/1
  freeze_cntr1/2(we) -> Delay6/1
  freeze_cntr1/1(addr) -> Delay3/1
  acc_core/2(valid) -> Delay1/1
  rst/1 -> acc_core/3(rst)
  we/1 -> acc_core/2(we)
  din/1 -> acc_core/1(din)
  Delay/1 -> bram/2, Gateway Out/1
  Constant/1 -> ctrl/1
  Delay1/1 -> Gateway Out1/1, Inverter/1, bram/3, Register/3
  Delay2/1 -> Logical/2
  Delay3/1 -> Gateway Out2/1, bram/1, Register/1
  Register/1 -> addr/1
  acc_core/3(empty) -> Delay4/1
  Logical/1 -> Concat/2
  Concat/1 -> done/1
  Delay4/1 -> Concat/1
  Delay6/1 -> acc_core/4(re)
  Delay5/1 -> Register/2

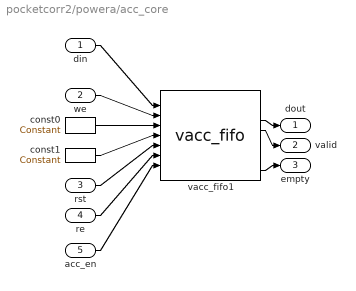
== system pocketcorr2/powera/acc_core ==
  din : Inport  Port=1  LatchInput=off
  we : Inport  Port=2  LatchInput=off
  rst : Inport  Port=3  LatchInput=off
  re : Inport  Port=4  LatchInput=off
  acc_en : Inport  Port=5  LatchInput=off
  const0 : xbsIndex_r3/Constant  const=0  equ=P=C  arith_type=Unsigned  n_bits=n_bits  bin_pt=bin_pt  opselect=C  inp2=PCIN>>17  opr=+  inp1=P  carry=CIN  iostate=0  explicit_period=on  period=1  dbl_ovrd=off
  const1 : xbsIndex_r3/Constant  const=0  equ=P=C  arith_type=Boolean  n_bits=1  bin_pt=0  opselect=C  inp2=PCIN>>17  opr=+  inp1=P  carry=CIN  iostate=0  explicit_period=on  period=1  dbl_ovrd=off
  vacc_fifo1 : correlator_library/vacc_fifo  vlen=vlen  n_bits=n_bits  bin_pt=bin_pt  add_latency=add_latency  arith_type=Unsigned  BitWidthIn=BitWidthIn  BinPtIn=BinPtIn  streams=streams  stream=1
      link override constant: equ=P=C  arith_type="Signed  (2's comp)"
  dout : Outport
  valid : Outport  Port=2
  empty : Outport  Port=3
  wires:
  din/1 -> vacc_fifo1/1
  we/1 -> vacc_fifo1/2
  const0/1 -> vacc_fifo1/3
  const1/1 -> vacc_fifo1/4
  rst/1 -> vacc_fifo1/5
  re/1 -> vacc_fifo1/6
  acc_en/1 -> vacc_fifo1/7
  vacc_fifo1/3 -> dout/1
  vacc_fifo1/4 -> valid/1
  vacc_fifo1/8 -> empty/1

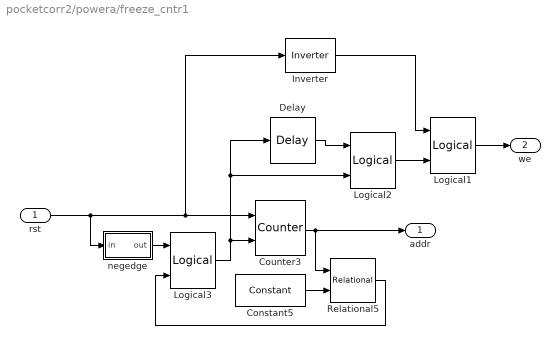
== system pocketcorr2/powera/freeze_cntr1 ==
  rst : Inport  Port=1  LatchInput=off
  Constant5 : xbsIndex_r3/Constant  const=2^CounterBits - 2  equ=P=C  arith_type=Unsigned  n_bits=CounterBits  bin_pt=0  opselect=C  inp2=PCIN>>17  opr=+  inp1=P  carry=CIN  iostate=0  explicit_period=off  period=1  dbl_ovrd=off
  Counter3 : xbsIndex_r3/Counter  cnt_type=Free Running  n_bits=CounterBits  bin_pt=0  arith_type=Unsigned  start_count=0  cnt_to=1023  cnt_by_val=1  operation=Up  explicit_period=on  period=1  load_pin=off  rst=on  en=on  dbl_ovrd=off  show_param=off  use_rpm=on  gen_core=off
      settings: xl_area=[0, 0, 0, 0, 0, 0, 0]
  Delay : xbsIndex_r3/Delay  latency=1  reg_retiming=off  explicit_period=off  period=1  en=off  accept_only_valid=off  init_zero=on  dbl_ovrd=off  show_param=off
      settings: xl_area=[0, 0, 0, 0, 0, 0, 0]
  Inverter : xbsIndex_r3/Inverter  latency=0  explicit_period=off  period=1  en=off  dbl_ovrd=off  show_param=off
      settings: xl_area=[0, 0, 0, 0, 0, 0, 0]
  Logical1 : xbsIndex_r3/Logical  logical_function=AND  inputs=2  precision=Full  arith_type=Unsigned  n_bits=8  bin_pt=2  align_bp=on  latency=0  explicit_period=off  period=1  en=off  dbl_ovrd=off  show_param=off
      settings: xl_area=[0, 0, 0, 0, 0, 0, 0]
  Logical2 : xbsIndex_r3/Logical  logical_function=OR  inputs=2  precision=Full  arith_type=Unsigned  n_bits=8  bin_pt=2  align_bp=on  latency=0  explicit_period=off  period=1  en=off  dbl_ovrd=off  show_param=off
      settings: xl_area=[0, 0, 0, 0, 0, 0, 0]
  Logical3 : xbsIndex_r3/Logical  logical_function=OR  inputs=2  precision=Full  arith_type=Unsigned  n_bits=8  bin_pt=2  align_bp=on  latency=0  explicit_period=off  period=1  en=off  dbl_ovrd=off  show_param=off
      settings: xl_area=[0, 0, 0, 0, 0, 0, 0]
  Relational5 : xbsIndex_r3/Relational  mode=a<b  latency=1  explicit_period=off  period=1  en=off  dbl_ovrd=off  show_param=off
      settings: xl_area=[0, 0, 0, 0, 0, 0, 0]
  negedge : Subsystem
  addr : Outport
  we : Outport  Port=2
  wires:
  Delay/1 -> Logical2/1
  Logical2/1 -> Logical1/2
  negedge/1(out) -> Logical3/1
  Relational5/1 -> Logical3/2
  Logical3/1 -> Delay/1, Logical2/2, Counter3/2
  Inverter/1 -> Logical1/1
  Logical1/1 -> we/1
  rst/1 -> negedge/1(in), Inverter/1, Counter3/1
  Constant5/1 -> Relational5/2
  Counter3/1 -> Relational5/1, addr/1

== system pocketcorr2/powera/posedge ==
  in : Inport  Port=1  LatchInput=off
  Delay : xbsIndex_r3/Delay  latency=1  reg_retiming=off  explicit_period=off  period=1  en=off  accept_only_valid=off  init_zero=on  dbl_ovrd=off  show_param=off
      settings: xl_area=[0, 0, 0, 0, 0, 0, 0]
  Inverter : xbsIndex_r3/Inverter  latency=0  explicit_period=off  period=1  en=off  dbl_ovrd=off  show_param=off
      settings: xl_area=[0, 0, 0, 0, 0, 0, 0]
  Logical : xbsIndex_r3/Logical  logical_function=AND  inputs=2  precision=Full  arith_type=Unsigned  n_bits=8  bin_pt=2  align_bp=on  latency=0  explicit_period=off  period=1  en=off  dbl_ovrd=off  show_param=off
      settings: xl_area=[0, 0, 0, 0, 0, 0, 0]
  out : Outport
  wires:
  Logical/1 -> out/1
  in/1 -> Logical/2, Delay/1
  Inverter/1 -> Logical/1
  Delay/1 -> Inverter/1

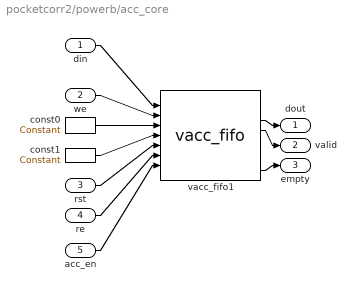
== system pocketcorr2/powerb/acc_core ==
  din : Inport  Port=1  LatchInput=off
  we : Inport  Port=2  LatchInput=off
  rst : Inport  Port=3  LatchInput=off
  re : Inport  Port=4  LatchInput=off
  acc_en : Inport  Port=5  LatchInput=off
  const0 : xbsIndex_r3/Constant  const=0  equ=P=C  arith_type=Unsigned  n_bits=n_bits  bin_pt=bin_pt  opselect=C  inp2=PCIN>>17  opr=+  inp1=P  carry=CIN  iostate=0  explicit_period=on  period=1  dbl_ovrd=off
  const1 : xbsIndex_r3/Constant  const=0  equ=P=C  arith_type=Boolean  n_bits=1  bin_pt=0  opselect=C  inp2=PCIN>>17  opr=+  inp1=P  carry=CIN  iostate=0  explicit_period=on  period=1  dbl_ovrd=off
  vacc_fifo1 : correlator_library/vacc_fifo  vlen=vlen  n_bits=n_bits  bin_pt=bin_pt  add_latency=add_latency  arith_type=Unsigned  BitWidthIn=BitWidthIn  BinPtIn=BinPtIn  streams=streams  stream=1
      link override constant: equ=P=C  arith_type=Unsigned
  dout : Outport
  valid : Outport  Port=2
  empty : Outport  Port=3
  wires:
  din/1 -> vacc_fifo1/1
  we/1 -> vacc_fifo1/2
  const0/1 -> vacc_fifo1/3
  const1/1 -> vacc_fifo1/4
  rst/1 -> vacc_fifo1/5
  re/1 -> vacc_fifo1/6
  acc_en/1 -> vacc_fifo1/7
  vacc_fifo1/3 -> dout/1
  vacc_fifo1/4 -> valid/1
  vacc_fifo1/8 -> empty/1

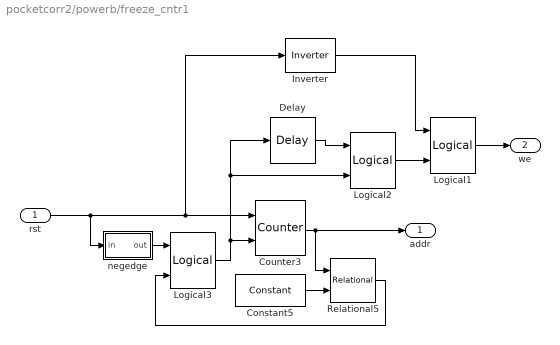
== system pocketcorr2/powerb/freeze_cntr1 ==
  rst : Inport  Port=1  LatchInput=off
  Constant5 : xbsIndex_r3/Constant  const=2^CounterBits - 2  equ=P=C  arith_type=Unsigned  n_bits=CounterBits  bin_pt=0  opselect=C  inp2=PCIN>>17  opr=+  inp1=P  carry=CIN  iostate=0  explicit_period=off  period=1  dbl_ovrd=off
  Counter3 : xbsIndex_r3/Counter  cnt_type=Free Running  n_bits=CounterBits  bin_pt=0  arith_type=Unsigned  start_count=0  cnt_to=1023  cnt_by_val=1  operation=Up  explicit_period=on  period=1  load_pin=off  rst=on  en=on  dbl_ovrd=off  show_param=off  use_rpm=on  gen_core=off
      settings: xl_area=[0, 0, 0, 0, 0, 0, 0]
  Delay : xbsIndex_r3/Delay  latency=1  reg_retiming=off  explicit_period=off  period=1  en=off  accept_only_valid=off  init_zero=on  dbl_ovrd=off  show_param=off
      settings: xl_area=[0, 0, 0, 0, 0, 0, 0]
  Inverter : xbsIndex_r3/Inverter  latency=0  explicit_period=off  period=1  en=off  dbl_ovrd=off  show_param=off
      settings: xl_area=[0, 0, 0, 0, 0, 0, 0]
  Logical1 : xbsIndex_r3/Logical  logical_function=AND  inputs=2  precision=Full  arith_type=Unsigned  n_bits=8  bin_pt=2  align_bp=on  latency=0  explicit_period=off  period=1  en=off  dbl_ovrd=off  show_param=off
      settings: xl_area=[0, 0, 0, 0, 0, 0, 0]
  Logical2 : xbsIndex_r3/Logical  logical_function=OR  inputs=2  precision=Full  arith_type=Unsigned  n_bits=8  bin_pt=2  align_bp=on  latency=0  explicit_period=off  period=1  en=off  dbl_ovrd=off  show_param=off
      settings: xl_area=[0, 0, 0, 0, 0, 0, 0]
  Logical3 : xbsIndex_r3/Logical  logical_function=OR  inputs=2  precision=Full  arith_type=Unsigned  n_bits=8  bin_pt=2  align_bp=on  latency=0  explicit_period=off  period=1  en=off  dbl_ovrd=off  show_param=off
      settings: xl_area=[0, 0, 0, 0, 0, 0, 0]
  Relational5 : xbsIndex_r3/Relational  mode=a<b  latency=1  explicit_period=off  period=1  en=off  dbl_ovrd=off  show_param=off
      settings: xl_area=[0, 0, 0, 0, 0, 0, 0]
  negedge : Subsystem
  addr : Outport
  we : Outport  Port=2
  wires:
  Delay/1 -> Logical2/1
  Logical2/1 -> Logical1/2
  negedge/1(out) -> Logical3/1
  Relational5/1 -> Logical3/2
  Logical3/1 -> Delay/1, Logical2/2, Counter3/2
  Inverter/1 -> Logical1/1
  Logical1/1 -> we/1
  rst/1 -> negedge/1(in), Inverter/1, Counter3/1
  Constant5/1 -> Relational5/2
  Counter3/1 -> Relational5/1, addr/1

== system pocketcorr2/powerb/posedge ==
  in : Inport  Port=1  LatchInput=off
  Delay : xbsIndex_r3/Delay  latency=1  reg_retiming=off  explicit_period=off  period=1  en=off  accept_only_valid=off  init_zero=on  dbl_ovrd=off  show_param=off
      settings: xl_area=[0, 0, 0, 0, 0, 0, 0]
  Inverter : xbsIndex_r3/Inverter  latency=0  explicit_period=off  period=1  en=off  dbl_ovrd=off  show_param=off
      settings: xl_area=[0, 0, 0, 0, 0, 0, 0]
  Logical : xbsIndex_r3/Logical  logical_function=AND  inputs=2  precision=Full  arith_type=Unsigned  n_bits=8  bin_pt=2  align_bp=on  latency=0  explicit_period=off  period=1  en=off  dbl_ovrd=off  show_param=off
      settings: xl_area=[0, 0, 0, 0, 0, 0, 0]
  out : Outport
  wires:
  Logical/1 -> out/1
  in/1 -> Logical/2, Delay/1
  Inverter/1 -> Logical/1
  Delay/1 -> Inverter/1

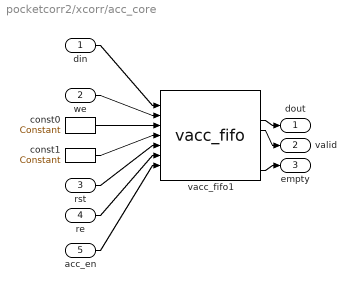
== system pocketcorr2/xcorr/acc_core ==
  din : Inport  Port=1  LatchInput=off
  we : Inport  Port=2  LatchInput=off
  rst : Inport  Port=3  LatchInput=off
  re : Inport  Port=4  LatchInput=off
  acc_en : Inport  Port=5  LatchInput=off
  const0 : xbsIndex_r3/Constant  const=0  equ=P=C  arith_type=Unsigned  n_bits=n_bits  bin_pt=bin_pt  opselect=C  inp2=PCIN>>17  opr=+  inp1=P  carry=CIN  iostate=0  explicit_period=on  period=1  dbl_ovrd=off
  const1 : xbsIndex_r3/Constant  const=0  equ=P=C  arith_type=Boolean  n_bits=1  bin_pt=0  opselect=C  inp2=PCIN>>17  opr=+  inp1=P  carry=CIN  iostate=0  explicit_period=on  period=1  dbl_ovrd=off
  vacc_fifo1 : correlator_library/vacc_fifo  vlen=vlen  n_bits=n_bits  bin_pt=bin_pt  add_latency=add_latency  arith_type=Unsigned  BitWidthIn=BitWidthIn  BinPtIn=BinPtIn  streams=streams  stream=1
      link override constant: equ=P=C  arith_type=Unsigned
  dout : Outport
  valid : Outport  Port=2
  empty : Outport  Port=3
  wires:
  din/1 -> vacc_fifo1/1
  we/1 -> vacc_fifo1/2
  const0/1 -> vacc_fifo1/3
  const1/1 -> vacc_fifo1/4
  rst/1 -> vacc_fifo1/5
  re/1 -> vacc_fifo1/6
  acc_en/1 -> vacc_fifo1/7
  vacc_fifo1/3 -> dout/1
  vacc_fifo1/4 -> valid/1
  vacc_fifo1/8 -> empty/1

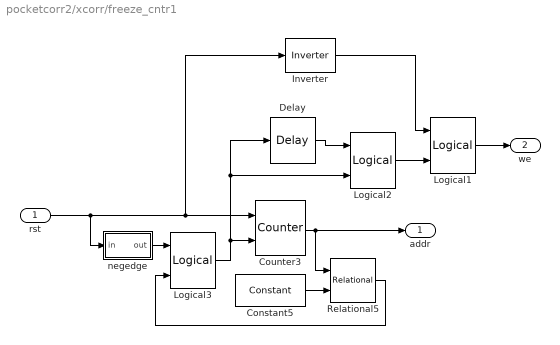
== system pocketcorr2/xcorr/freeze_cntr1 ==
  rst : Inport  Port=1  LatchInput=off
  Constant5 : xbsIndex_r3/Constant  const=2^CounterBits - 2  equ=P=C  arith_type=Unsigned  n_bits=CounterBits  bin_pt=0  opselect=C  inp2=PCIN>>17  opr=+  inp1=P  carry=CIN  iostate=0  explicit_period=off  period=1  dbl_ovrd=off
  Counter3 : xbsIndex_r3/Counter  cnt_type=Free Running  n_bits=CounterBits  bin_pt=0  arith_type=Unsigned  start_count=0  cnt_to=1023  cnt_by_val=1  operation=Up  explicit_period=on  period=1  load_pin=off  rst=on  en=on  dbl_ovrd=off  show_param=off  use_rpm=on  gen_core=off
      settings: xl_area=[0, 0, 0, 0, 0, 0, 0]
  Delay : xbsIndex_r3/Delay  latency=1  reg_retiming=off  explicit_period=off  period=1  en=off  accept_only_valid=off  init_zero=on  dbl_ovrd=off  show_param=off
      settings: xl_area=[0, 0, 0, 0, 0, 0, 0]
  Inverter : xbsIndex_r3/Inverter  latency=0  explicit_period=off  period=1  en=off  dbl_ovrd=off  show_param=off
      settings: xl_area=[0, 0, 0, 0, 0, 0, 0]
  Logical1 : xbsIndex_r3/Logical  logical_function=AND  inputs=2  precision=Full  arith_type=Unsigned  n_bits=8  bin_pt=2  align_bp=on  latency=0  explicit_period=off  period=1  en=off  dbl_ovrd=off  show_param=off
      settings: xl_area=[0, 0, 0, 0, 0, 0, 0]
  Logical2 : xbsIndex_r3/Logical  logical_function=OR  inputs=2  precision=Full  arith_type=Unsigned  n_bits=8  bin_pt=2  align_bp=on  latency=0  explicit_period=off  period=1  en=off  dbl_ovrd=off  show_param=off
      settings: xl_area=[0, 0, 0, 0, 0, 0, 0]
  Logical3 : xbsIndex_r3/Logical  logical_function=OR  inputs=2  precision=Full  arith_type=Unsigned  n_bits=8  bin_pt=2  align_bp=on  latency=0  explicit_period=off  period=1  en=off  dbl_ovrd=off  show_param=off
      settings: xl_area=[0, 0, 0, 0, 0, 0, 0]
  Relational5 : xbsIndex_r3/Relational  mode=a<b  latency=1  explicit_period=off  period=1  en=off  dbl_ovrd=off  show_param=off
      settings: xl_area=[0, 0, 0, 0, 0, 0, 0]
  negedge : Subsystem
  addr : Outport
  we : Outport  Port=2
  wires:
  Counter3/1 -> addr/1, Relational5/1
  Constant5/1 -> Relational5/2
  rst/1 -> Counter3/1, Inverter/1, negedge/1(in)
  Logical1/1 -> we/1
  Inverter/1 -> Logical1/1
  Logical3/1 -> Counter3/2, Logical2/2, Delay/1
  Relational5/1 -> Logical3/2
  negedge/1(out) -> Logical3/1
  Logical2/1 -> Logical1/2
  Delay/1 -> Logical2/1
